simulink model "navion_simulation_Gramajo_yaw_rate_feedback"  (Simulink 8.7)
settings: Solver=ode45  StartTime=0.0  StopTime=20  MaxStep=0.1  RelTol=1e-3
PreLoadFcn:
  | aero1=datcomimport('NavionOut.out');
  | load bank_turn.mat
  | load elevator.mat
  | modify
values from neighbouring files (symbols this model uses):
  aileron = [-45 -40 -35 -30 -25 -20 -15 -10 -5 0 5 10 ... (19 elements, 1x19)]    [bank_turn.mat]    (also in calc_bank_turn.m = -45:5:45)
  delCl = [-0.189280957379 -0.179943445881 -0.170605934382 -0.161268422884 -0.151930911386 -0.142593399888 -0.13325588839 -0.123918376892 -0.114580865393 -0.105243353895 -0.0959058423971 -0.0865683308989 ... (361 elements, 19x19)]    [bank_turn.mat]
  delCn = [0.0592975613365 0.0530143760293 0.0467311907221 0.040448005415 0.0341648201078 0.0278816348006 0.0215984494934 0.0153152641863 0.00903207887907 0.00274889357189 -0.00353429173529 -0.00981747704247 ... (361 elements, 19x19)]    [bank_turn.mat]
  delCy = [-0.123307511653 -0.109606677025 -0.0959058423971 -0.0822050077689 -0.0685041731408 -0.0548033385126 -0.0411025038845 -0.0274016692563 -0.0137008346282 0 0.0137008346282 0.0274016692563 ... (19 elements, 1x19)]    [bank_turn.mat]
  dt = 5    [search_and_coverage.m]    (also in search_and_coverage_multiple_turn_durations.m = Turn_durations(ii); search_and_coverage_time_constraint.m = 13)
  rudder = [-45 -40 -35 -30 -25 -20 -15 -10 -5 0 5 10 ... (19 elements, 1x19)]    [bank_turn.mat]    (also in calc_bank_turn.m = -45:5:45)
  V_mass = 5    [search_and_coverage.m]    (also in search_and_coverage_multiple_turn_durations.m; search_and_coverage_time_constraint.m)
  Velocity = vel    [RHC_opt.m]    (also in RHC_opt_mod_algo.m; search_and_coverage.m = sqrt(2*Weight/(rho*W_area)*(1/CL)); search_and_coverage_multiple_turn_durations.m = sqrt(2*Weight/(rho*W_area)*(1/CL)); search_and_coverage_time_constraint.m = sqrt(2*Weight/(rho*W_area)*(1/CL)))
undefined symbols (not defined in the file or in its folder): alpha_table, delCD, delCL, delCm, delE, desired_omega
libraries: aerolibasang x4, simulink x3, aerolibtransform2 x2, aerolib6dof2 x1, aerolibatmos2 x1, aerolibadyn x1, aerolibutil x1
settings Model: Creator=ggramajo  LastModifiedBy=ggramajo
settings DataIOCC: LimitDataPoints=off  SaveFormat=Structure
settings DebuggingCC: AlgebraicLoopMsg=none  UnderspecifiedInitializationDetection=Simplified  MergeDetectMultiDrivingBlocksExec=error
settings HardwareCC: ProdBitPerPointer=64  ProdLargestAtomicFloat=Float  ProdIntDivRoundTo=Zero  ProdEndianess=LittleEndian  ProdWordSize=64  ProdHWDeviceType=Intel->x86-64 (Windows64)
settings ModelReferenceCC: PropagateSignalLabelsOutOfModel=on
settings ConfigComp: CovModelRefEnable=off

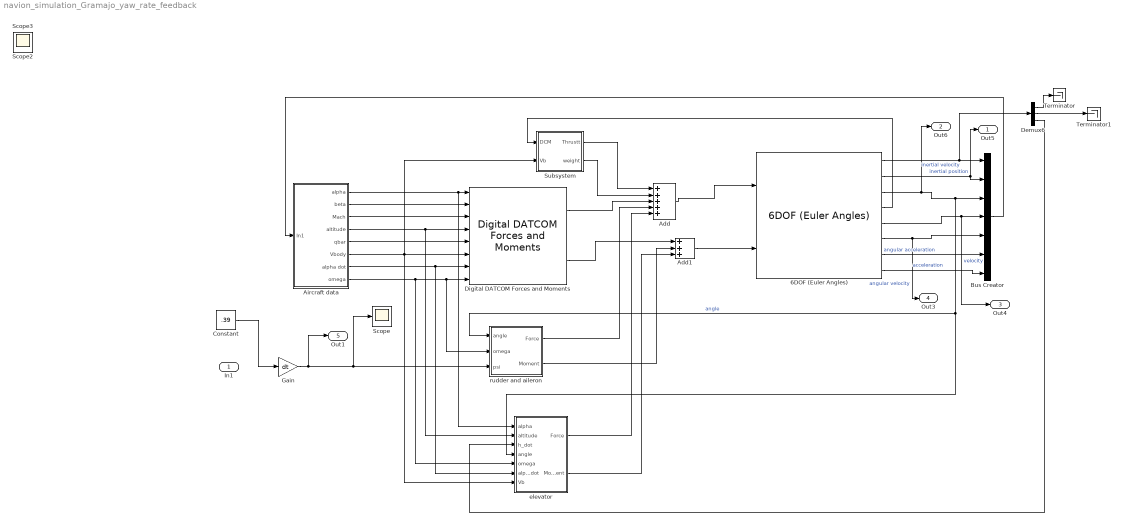
== system navion_simulation_Gramajo_yaw_rate_feedback ==
  In1 : Inport
  6DOF (Euler Angles) : aerolib6dof2/6DOF (Euler Angles)  units=Metric (MKS)  mtype=Fixed  rep=Euler Angles  xme_0=[0 0 -121]  Vm_0=[28 0 0]  eul_0=[0 0 0]  pm_0=[0 0 0]  mass_0=V_mass  mass_e=0.5  mass_f=2.0  inertia=[.057 0 0;0 .163 0;0 0 .192]  inertia_e=eye(3)  inertia_f=2*eye(3)  k_quat=1.0  vre_flag=on
  Add : Sum  Inputs=+++++
  Add1 : Sum  Inputs=+++
  "Aircraft data " : Subsystem
  Bus Creator : BusCreator  Inputs=7
  Constant : Constant  Value=.39
  Demux6 : Demux  Outputs=3
  Digital DATCOM Forces and Moments : aerolibadyn/Digital DATCOM Forces and Moments  units=Metric (MKS)  dcase=aero1{1}  fmode=Body  buildno=0  imethod=Linear  emethod=Linear  rmethod=Linear Extrapolation  action=None
  Gain : Gain  Gain=dt
  Scope : Scope
  Subsystem : Subsystem
  Terminator : Terminator
  Terminator1 : Terminator
  elevator : Subsystem
  rudder and aileron : Subsystem
  Out5 : Outport
  Out6 : Outport  Port=2
  Out4 : Outport  Port=3
  Out3 : Outport  Port=4
  Out1 : Outport  Port=5
  Scope2 : Scope
  Scope3 : Scope
  wires:
  "Aircraft data "/3(Mach) -> Digital DATCOM Forces and Moments/3
  "Aircraft data "/5("qbar ") -> Digital DATCOM Forces and Moments/5
  "Aircraft data "/6(Vbody) -> elevator/7(Vb), Subsystem/2("Vb "), Digital DATCOM Forces and Moments/6
  "Aircraft data "/1(alpha) -> elevator/1(alpha), Digital DATCOM Forces and Moments/1
  Add/1 -> 6DOF (Euler Angles)/1
  Add1/1 -> 6DOF (Euler Angles)/2
  6DOF (Euler Angles)/1 -> Demux6/1, Bus Creator/1  "inertial velocity"
  6DOF (Euler Angles)/2 -> Bus Creator/2, Out5/1  "inertial position"
  6DOF (Euler Angles)/3 -> Out6/1, elevator/4(angle), rudder and aileron/1(angle), Bus Creator/3  "angle"
  6DOF (Euler Angles)/5 -> Out4/1, Bus Creator/4  "velocity"
  6DOF (Euler Angles)/6 -> Out3/1, Bus Creator/5  "angular velocity"
  6DOF (Euler Angles)/7 -> Bus Creator/6  "angular acceleration"
  6DOF (Euler Angles)/8 -> Bus Creator/7  "acceleration"
  Bus Creator/1 -> "Aircraft data "/1(In1)
  "Aircraft data "/2(beta) -> Digital DATCOM Forces and Moments/2
  Digital DATCOM Forces and Moments/1 -> Add/3
  "Aircraft data "/7("alpha dot ") -> elevator/6(alpha_dot), Digital DATCOM Forces and Moments/7
  "Aircraft data "/8(omega) -> elevator/5(omega), rudder and aileron/2(omega), Digital DATCOM Forces and Moments/8
  Digital DATCOM Forces and Moments/2 -> Add1/1
  "Aircraft data "/4(altitude) -> elevator/2(altitude), Digital DATCOM Forces and Moments/4
  6DOF (Euler Angles)/4 -> Subsystem/1(DCM)
  Demux6/3 -> elevator/3(h_dot)
  Subsystem/1("Thrustt ") -> Add/1
  Subsystem/2(weight) -> Add/2
  elevator/1(Force) -> Add/5
  elevator/2(Moment) -> Add1/3
  rudder and aileron/1(Force) -> Add/4
  rudder and aileron/2(Moment) -> Add1/2
  Demux6/1 -> Terminator/1
  Demux6/2 -> Terminator1/1
  Gain/1 -> Scope/1, rudder and aileron/3(psi), Out1/1
  Constant/1 -> Gain/1

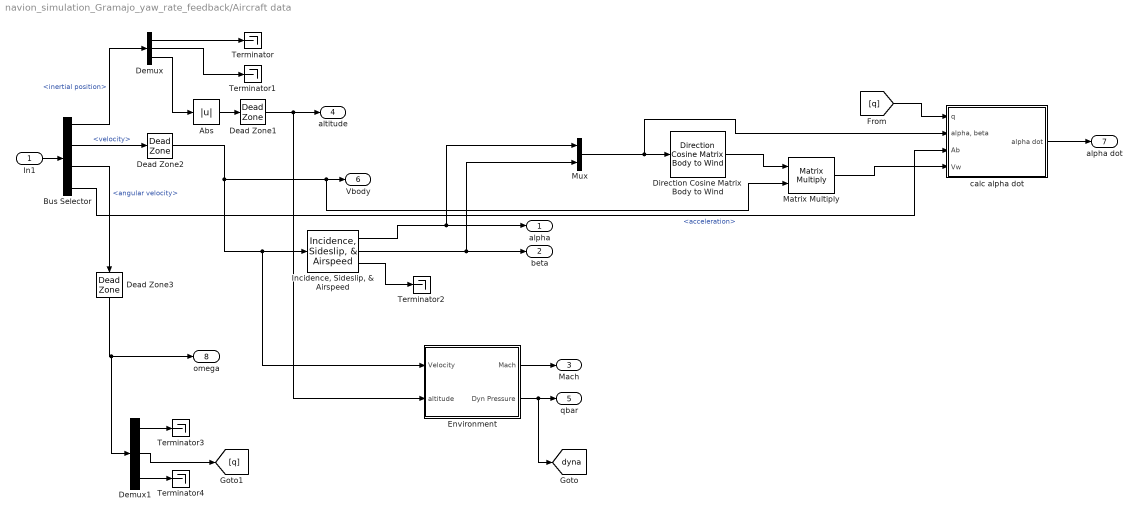
== system navion_simulation_Gramajo_yaw_rate_feedback/Aircraft data  ==
  In1 : Inport
  Abs : Abs
  Bus Selector : BusSelector  OutputSignals=inertial position,velocity,angular velocity,acceleration
  Dead Zone1 : DeadZone  LowerValue=-0.001  UpperValue=0.001  SaturateOnIntegerOverflow=on
  Dead Zone2 : DeadZone  LowerValue=-0.001  UpperValue=0.001  SaturateOnIntegerOverflow=on
  Dead Zone3 : DeadZone  LowerValue=-0.001  UpperValue=0.001  SaturateOnIntegerOverflow=on
  Demux : Demux  Outputs=3
  Demux1 : Demux  Outputs=3
  Direction Cosine Matrix Body to Wind : aerolibtransform2/Direction Cosine Matrix Body to Wind
  Environment : Subsystem
  "Incidence, Sideslip, & Airspeed" : aerolibasang/Incidence, Sideslip, & Airspeed
  Matrix Multiply : Product  Multiplication=Matrix(*)
  Mux : Mux  Inputs=2
  Terminator{,1..4} (5 alike) : Terminator
  calc alpha dot : Subsystem
  alpha : Outport
  beta : Outport  Port=2
  Mach : Outport  Port=3
  altitude : Outport  Port=4
  "qbar " : Outport  Port=5
  Vbody : Outport  Port=6
  "alpha dot " : Outport  Port=7
  omega : Outport  Port=8
  tag scope: dyna=global
  wires:
  In1/1 -> Bus Selector/1
  Bus Selector/1 -> Demux/1  "<inertial position>"
  Demux/1 -> Terminator/1
  Demux/3 -> Abs/1
  Demux/2 -> Terminator1/1
  Bus Selector/2 -> Dead Zone2/1  "<velocity>"
  "Incidence, Sideslip, & Airspeed"/1 -> Mux/1, alpha/1
  "Incidence, Sideslip, & Airspeed"/2 -> Mux/2, beta/1
  "Incidence, Sideslip, & Airspeed"/3 -> Terminator2/1
  Dead Zone1/1 -> Environment/2(altitude), altitude/1
  Abs/1 -> Dead Zone1/1
  Environment/1(Mach) -> Mach/1
  Environment/2(Dyn Pressure) -> [dyna], "qbar "/1
  Mux/1 -> calc alpha dot/2("alpha, beta"), Direction Cosine Matrix Body to Wind/1
  Bus Selector/3 -> Dead Zone3/1  "<angular velocity>"
  Direction Cosine Matrix Body to Wind/1 -> Matrix Multiply/1
  Bus Selector/4 -> calc alpha dot/3("Ab ")  "<acceleration>"
  [q] -> calc alpha dot/1("q ")
  Demux1/1 -> Terminator3/1
  Demux1/2 -> [q]
  calc alpha dot/1("alpha dot ") -> "alpha dot "/1
  Matrix Multiply/1 -> calc alpha dot/4("Vw ")
  Demux1/3 -> Terminator4/1
  Dead Zone2/1 -> Environment/1("Velocity "), "Incidence, Sideslip, & Airspeed"/1, Matrix Multiply/2, Vbody/1
  Dead Zone3/1 -> omega/1, Demux1/1

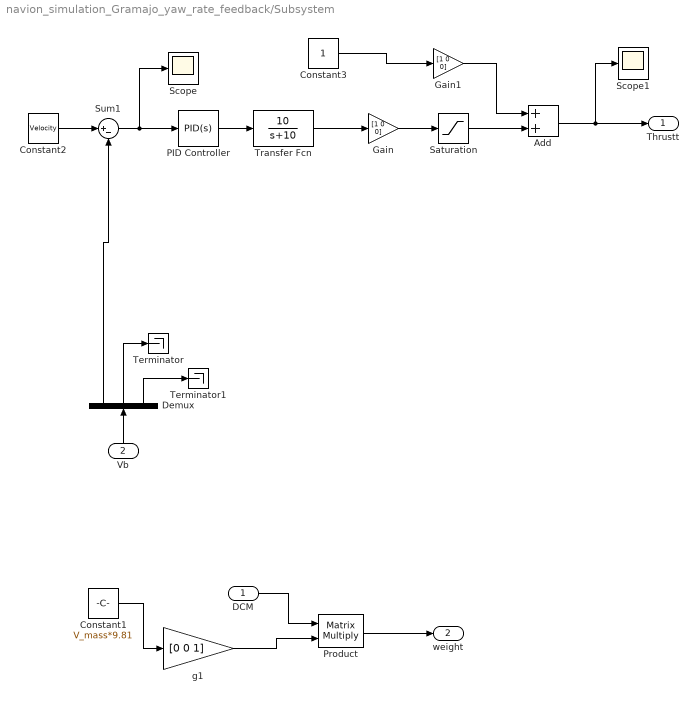
== system navion_simulation_Gramajo_yaw_rate_feedback/Subsystem ==
  DCM : Inport
  "Vb " : Inport  Port=2
  Add : Sum
  Constant1 : Constant  Value=V_mass*9.81
  Constant2 : Constant  Value=Velocity
  Constant3 : Constant
  Demux : Demux  Outputs=3
  Gain : Gain  Gain=[1 0 0]
  Gain1 : Gain  Gain=[1 0 0]
  PID Controller : simulink/Continuous/PID Controller  Controller=PID  TimeDomain=Continuous-time  SampleTime=-1  IntegratorMethod=Forward Euler  FilterMethod=Forward Euler  Form=Parallel  UseFilter=on  ControllerParametersSource=internal  P=1378.85680869118  I=7872.63938553885  D=41.0333927112897  N=486.626215957967  InitialConditionSource=internal  InitialConditionForIntegrator=0  InitialConditionForFilter=0  ExternalReset=none  LimitOutput=off  UpperSaturationLimit=inf  LowerSaturationLimit=-inf  LinearizeAsGain=on  AntiWindupMode=none  Kb=1  TrackingMode=off  Kt=1  PParamMin=[]  PParamMax=[]  IParamMin=[]  IParamMax=[]  DParamMin=[]  DParamMax=[]  NParamMin=[]  NParamMax=[]  KbParamMin=[]  KbParamMax=[]  KtParamMin=[]  KtParamMax=[]  POutMin=[]  POutMax=[]  IOutMin=[]  IOutMax=[]  DOutMin=[]  DOutMax=[]  NOutMin=[]  NOutMax=[]  KbOutMin=[]  KbOutMax=[]  KtOutMin=[]  KtOutMax=[]  IntegratorOutMin=[]  IntegratorOutMax=[]  FilterOutMin=[]  FilterOutMax=[]  SumOutMin=[]  SumOutMax=[]  SumI1OutMin=[]  SumI1OutMax=[]  SumI2OutMin=[]  SumI2OutMax=[]  SumI3OutMin=[]  SumI3OutMax=[]  SumDOutMin=[]  SumDOutMax=[]  SaturationOutMin=[]  SaturationOutMax=[]  IntegratorContinuousStateAttributes=''  IntegratorStateMustResolveToSignalObject=off  IntegratorRTWStateStorageClass=Auto  FilterContinuousStateAttributes=''  FilterStateMustResolveToSignalObject=off  FilterRTWStateStorageClass=Auto  DifferentiatorICPrevScaledInput=0  DifferentiatorOutMin=[]  DifferentiatorOutMax=[]
  Product : Product  Multiplication=Matrix(*)  SaturateOnIntegerOverflow=on  InputSameDT=on  OutDataTypeStr=Inherit: Same as first input
  Saturation : Saturate  UpperLimit=5  LowerLimit=-1
  Scope : Scope
  Scope1 : Scope
  Sum1 : Sum  Inputs=|+-
  Terminator : Terminator
  Terminator1 : Terminator
  Transfer Fcn : TransferFcn  Numerator=[10]  Denominator=[1 10]
  g1 : Gain  Gain=[0 0 1]  SaturateOnIntegerOverflow=on  OutDataTypeStr=Inherit: Same as input  ParamDataTypeStr=Inherit: Same as input
  "Thrustt " : Outport
  weight : Outport  Port=2
  wires:
  Constant2/1 -> Sum1/1
  "Vb "/1 -> Demux/1
  Demux/2 -> Terminator/1
  Demux/3 -> Terminator1/1
  Transfer Fcn/1 -> Gain/1
  Demux/1 -> Sum1/2
  Sum1/1 -> Scope/1, PID Controller/1
  Constant1/1 -> g1/1
  DCM/1 -> Product/1
  g1/1 -> Product/2
  Product/1 -> weight/1
  PID Controller/1 -> Transfer Fcn/1
  Gain/1 -> Saturation/1
  Constant3/1 -> Gain1/1
  Gain1/1 -> Add/1
  Add/1 -> Scope1/1, "Thrustt "/1
  Saturation/1 -> Add/2

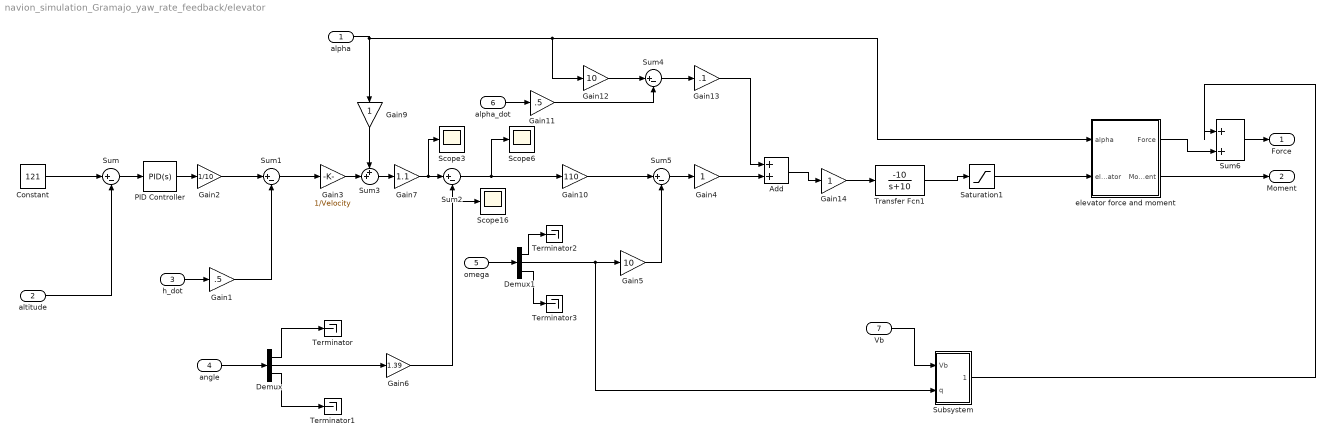
== system navion_simulation_Gramajo_yaw_rate_feedback/elevator ==
  alpha : Inport
  altitude : Inport  Port=2
  h_dot : Inport  Port=3
  angle : Inport  Port=4
  omega : Inport  Port=5
  alpha_dot : Inport  Port=6
  Vb : Inport  Port=7
  Add : Sum
  Constant : Constant  Value=121
  Demux : Demux  Outputs=3
  Demux1 : Demux  Outputs=3
  Gain1 : Gain  Gain=.5
  Gain10 : Gain  Gain=110
  Gain11 : Gain  Gain=.5
  Gain12 : Gain  Gain=10
  Gain13 : Gain  Gain=.1
  Gain14 : Gain
  Gain2 : Gain  Gain=1/10
  Gain3 : Gain  Gain=1/Velocity
  Gain4 : Gain
  Gain5 : Gain  Gain=10
  Gain6 : Gain  Gain=1.39
  Gain7 : Gain  Gain=1.1
  Gain9 : Gain
  PID Controller : simulink/Continuous/PID Controller  Controller=PID  TimeDomain=Continuous-time  SampleTime=-1  IntegratorMethod=Forward Euler  FilterMethod=Forward Euler  Form=Parallel  UseFilter=on  ControllerParametersSource=internal  P=27.8572060055225  I=30.4447135032815  D=6.28354456949659  N=474.535862872723  InitialConditionSource=internal  InitialConditionForIntegrator=0  InitialConditionForFilter=0  ExternalReset=none  LimitOutput=off  UpperSaturationLimit=inf  LowerSaturationLimit=-inf  LinearizeAsGain=on  AntiWindupMode=none  Kb=1  TrackingMode=off  Kt=1  PParamMin=[]  PParamMax=[]  IParamMin=[]  IParamMax=[]  DParamMin=[]  DParamMax=[]  NParamMin=[]  NParamMax=[]  KbParamMin=[]  KbParamMax=[]  KtParamMin=[]  KtParamMax=[]  POutMin=[]  POutMax=[]  IOutMin=[]  IOutMax=[]  DOutMin=[]  DOutMax=[]  NOutMin=[]  NOutMax=[]  KbOutMin=[]  KbOutMax=[]  KtOutMin=[]  KtOutMax=[]  IntegratorOutMin=[]  IntegratorOutMax=[]  FilterOutMin=[]  FilterOutMax=[]  SumOutMin=[]  SumOutMax=[]  SumI1OutMin=[]  SumI1OutMax=[]  SumI2OutMin=[]  SumI2OutMax=[]  SumI3OutMin=[]  SumI3OutMax=[]  SumDOutMin=[]  SumDOutMax=[]  SaturationOutMin=[]  SaturationOutMax=[]  IntegratorContinuousStateAttributes=''  IntegratorStateMustResolveToSignalObject=off  IntegratorRTWStateStorageClass=Auto  FilterContinuousStateAttributes=''  FilterStateMustResolveToSignalObject=off  FilterRTWStateStorageClass=Auto  DifferentiatorICPrevScaledInput=0  DifferentiatorOutMin=[]  DifferentiatorOutMax=[]
  Saturation1 : Saturate  UpperLimit=20  LowerLimit=-30
  Scope16 : Scope
  Scope3 : Scope
  Scope6 : Scope
  Subsystem : Subsystem
  Sum{,1..2,4..5} (5 alike) : Sum  Inputs=|+-
  Sum3 : Sum  Inputs=++|
  Sum6 : Sum  Inputs=|++
  Terminator{,1..3} (4 alike) : Terminator
  Transfer Fcn1 : TransferFcn  Numerator=[-10]  Denominator=[1 10]
  "elevator force and moment " : Subsystem
  Force : Outport
  Moment : Outport  Port=2
  wires:
  "elevator force and moment "/2(Moment) -> Moment/1
  Constant/1 -> Sum/1
  altitude/1 -> Sum/2
  h_dot/1 -> Gain1/1
  Saturation1/1 -> "elevator force and moment "/2(elevator)
  angle/1 -> Demux/1
  Demux/1 -> Terminator/1
  Demux/3 -> Terminator1/1
  omega/1 -> Demux1/1
  Sum5/1 -> Gain4/1
  Gain5/1 -> Sum5/2
  Sum2/1 -> Scope6/1, Gain10/1
  Gain1/1 -> Sum1/2
  Demux/2 -> Gain6/1
  Demux1/1 -> Terminator2/1
  Demux1/3 -> Terminator3/1
  Demux1/2 -> Gain5/1, Subsystem/2(q)
  Gain6/1 -> Scope16/1, Sum2/2
  Gain3/1 -> Sum3/2
  alpha/1 -> Gain12/1, "elevator force and moment "/1(alpha), Gain9/1
  Gain9/1 -> Sum3/1
  Sum1/1 -> Gain3/1
  Transfer Fcn1/1 -> Saturation1/1
  Sum/1 -> PID Controller/1
  Gain2/1 -> Sum1/1
  Gain10/1 -> Sum5/1
  Add/1 -> Gain14/1
  Gain4/1 -> Add/2
  Sum4/1 -> Gain13/1
  alpha_dot/1 -> Gain11/1
  Gain11/1 -> Sum4/2
  Gain12/1 -> Sum4/1
  Gain13/1 -> Add/1
  Gain14/1 -> Transfer Fcn1/1
  Sum3/1 -> Gain7/1
  Gain7/1 -> Scope3/1, Sum2/1
  PID Controller/1 -> Gain2/1
  Vb/1 -> Subsystem/1(Vb)
  Sum6/1 -> Force/1
  "elevator force and moment "/1(Force) -> Sum6/2
  Subsystem/1(CLq) -> Sum6/1

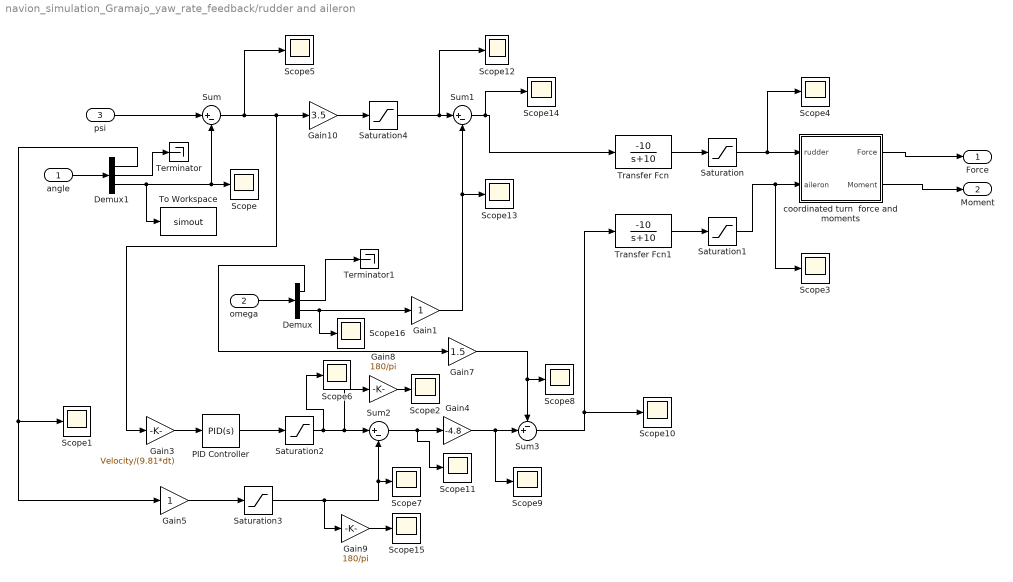
== system navion_simulation_Gramajo_yaw_rate_feedback/rudder and aileron ==
  angle : Inport
  omega : Inport  Port=2
  psi : Inport  Port=3
  Demux : Demux  Outputs=3
  Demux1 : Demux  Outputs=3
  Gain1 : Gain
  Gain10 : Gain  Gain=3.5
  Gain3 : Gain  Gain=Velocity/(9.81*dt)
  Gain4 : Gain  Gain=-4.8
  Gain5 : Gain
  Gain7 : Gain  Gain=1.5
  Gain8 : Gain  Gain=180/pi
  Gain9 : Gain  Gain=180/pi
  PID Controller : simulink/Continuous/PID Controller  Controller=PID  TimeDomain=Continuous-time  SampleTime=-1  IntegratorMethod=Forward Euler  FilterMethod=Forward Euler  Form=Parallel  UseFilter=on  ControllerParametersSource=internal  P=15.0986911644413  I=0.176703988972368  D=3.35005448489008  N=153.250185887762  InitialConditionSource=internal  InitialConditionForIntegrator=0  InitialConditionForFilter=0  ExternalReset=none  LimitOutput=off  UpperSaturationLimit=inf  LowerSaturationLimit=-inf  LinearizeAsGain=on  AntiWindupMode=none  Kb=1  TrackingMode=off  Kt=1  PParamMin=[]  PParamMax=[]  IParamMin=[]  IParamMax=[]  DParamMin=[]  DParamMax=[]  NParamMin=[]  NParamMax=[]  KbParamMin=[]  KbParamMax=[]  KtParamMin=[]  KtParamMax=[]  POutMin=[]  POutMax=[]  IOutMin=[]  IOutMax=[]  DOutMin=[]  DOutMax=[]  NOutMin=[]  NOutMax=[]  KbOutMin=[]  KbOutMax=[]  KtOutMin=[]  KtOutMax=[]  IntegratorOutMin=[]  IntegratorOutMax=[]  FilterOutMin=[]  FilterOutMax=[]  SumOutMin=[]  SumOutMax=[]  SumI1OutMin=[]  SumI1OutMax=[]  SumI2OutMin=[]  SumI2OutMax=[]  SumI3OutMin=[]  SumI3OutMax=[]  SumDOutMin=[]  SumDOutMax=[]  SaturationOutMin=[]  SaturationOutMax=[]  IntegratorContinuousStateAttributes=''  IntegratorStateMustResolveToSignalObject=off  IntegratorRTWStateStorageClass=Auto  FilterContinuousStateAttributes=''  FilterStateMustResolveToSignalObject=off  FilterRTWStateStorageClass=Auto  DifferentiatorICPrevScaledInput=0  DifferentiatorOutMin=[]  DifferentiatorOutMax=[]
  Saturation : Saturate  UpperLimit=15  LowerLimit=-15
  Saturation1 : Saturate  UpperLimit=20  LowerLimit=-20
  Saturation2 : Saturate  UpperLimit=.8411  LowerLimit=-.8411
  Saturation3 : Saturate  UpperLimit=.8411  LowerLimit=-.8411
  Saturation4 : Saturate  UpperLimit=1.5*desired_omega  LowerLimit=-1.5*abs(desired_omega)
  Scope{,1..16} (17 alike) : Scope
  Sum : Sum  Inputs=|+-
  Sum1 : Sum  Inputs=|+-
  Sum2 : Sum  Inputs=|+-
  Sum3 : Sum  Inputs=-+|
  Terminator : Terminator
  Terminator1 : Terminator
  To Workspace : ToWorkspace  VariableName=simout  SaveFormat=Structure With Time  SampleTime=-1
  Transfer Fcn : TransferFcn  Numerator=[-10]  Denominator=[1 10]
  Transfer Fcn1 : TransferFcn  Numerator=[-10]  Denominator=[1 10]
  "coordinated turn  force and moments  " : Subsystem
  Force : Outport
  Moment : Outport  Port=2
  wires:
  "coordinated turn  force and moments  "/1(Force) -> Force/1
  "coordinated turn  force and moments  "/2(Moment) -> Moment/1
  Transfer Fcn/1 -> Saturation/1
  Saturation/1 -> Scope4/1, "coordinated turn  force and moments  "/1(rudder)
  omega/1 -> Demux/1
  angle/1 -> Demux1/1
  Demux1/3 -> To Workspace/1, Scope/1, Sum/2
  Saturation1/1 -> Scope3/1, "coordinated turn  force and moments  "/2(aileron)
  Sum3/1 -> Scope10/1, Transfer Fcn1/1
  Sum1/1 -> Scope14/1, Transfer Fcn/1
  Demux1/1 -> Scope1/1, Gain5/1
  Demux1/2 -> Terminator/1
  Sum2/1 -> Scope11/1, Gain4/1
  Gain5/1 -> Saturation3/1
  PID Controller/1 -> Saturation2/1
  Demux/1 -> Gain7/1
  Gain4/1 -> Scope9/1, Sum3/2
  Gain7/1 -> Scope8/1, Sum3/1
  Transfer Fcn1/1 -> Saturation1/1
  Demux/2 -> Terminator1/1
  Gain3/1 -> PID Controller/1
  Sum/1 -> Gain3/1, Gain10/1, Scope5/1
  psi/1 -> Sum/1
  Gain1/1 -> Scope13/1, Sum1/2
  Gain8/1 -> Scope2/1
  Saturation2/1 -> Scope6/1, Gain8/1, Sum2/1
  Gain9/1 -> Scope15/1
  Saturation3/1 -> Gain9/1, Scope7/1, Sum2/2
  Demux/3 -> Gain1/1, Scope16/1
  Gain10/1 -> Saturation4/1
  Saturation4/1 -> Scope12/1, Sum1/1

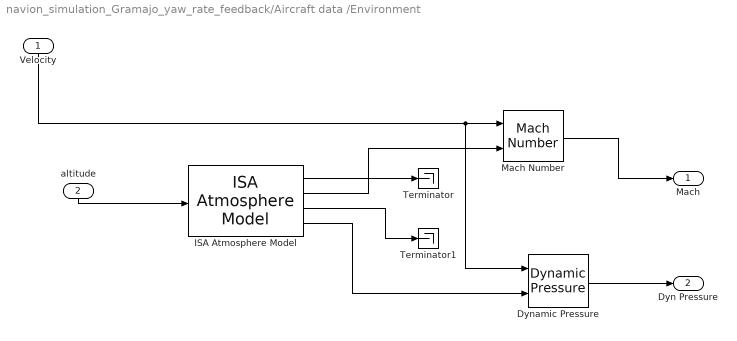
== system navion_simulation_Gramajo_yaw_rate_feedback/Aircraft data /Environment ==
  "Velocity " : Inport
  altitude : Inport  Port=2
  Dynamic Pressure : aerolibasang/Dynamic Pressure
  ISA Atmosphere Model : aerolibatmos2/ISA Atmosphere Model  custom=off  g=9.80665  gamma=1.4  R=287.0531  L=0.0065  h_trop=11000  h_strat=20000  rho0=1.225  P0=101325  T0=288.15  h0=0
  Mach Number : aerolibasang/Mach Number
  Terminator : Terminator
  Terminator1 : Terminator
  Mach : Outport
  Dyn Pressure : Outport  Port=2
  wires:
  Mach Number/1 -> Mach/1
  altitude/1 -> ISA Atmosphere Model/1
  ISA Atmosphere Model/2 -> Mach Number/2
  ISA Atmosphere Model/4 -> Dynamic Pressure/2
  ISA Atmosphere Model/1 -> Terminator/1
  ISA Atmosphere Model/3 -> Terminator1/1
  "Velocity "/1 -> Dynamic Pressure/1, Mach Number/1
  Dynamic Pressure/1 -> Dyn Pressure/1

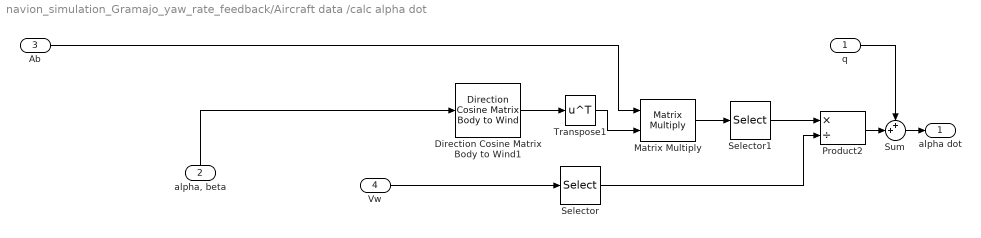
== system navion_simulation_Gramajo_yaw_rate_feedback/Aircraft data /calc alpha dot ==
  "q " : Inport
  "alpha, beta" : Inport  Port=2
  "Ab " : Inport  Port=3
  "Vw " : Inport  Port=4
  Direction Cosine Matrix Body to Wind1 : aerolibtransform2/Direction Cosine Matrix Body to Wind
  Matrix Multiply : Product  Multiplication=Matrix(*)
  Product2 : Product  Inputs=*/  SaturateOnIntegerOverflow=on  InputSameDT=on  OutDataTypeStr=Inherit: Same as first input
  Selector : Selector  InputPortWidth=3  IndexOptions=Index vector (dialog)  Indices=[1]  OutputSizes=1
  Selector1 : Selector  InputPortWidth=3  IndexOptions=Index vector (dialog)  Indices=[3]  OutputSizes=1
  Sum : Sum  Inputs=++|
  Transpose1 : Math  Operator=transpose  SaturateOnIntegerOverflow=on
  "alpha dot " : Outport
  wires:
  "Vw "/1 -> Selector/1
  Direction Cosine Matrix Body to Wind1/1 -> Transpose1/1
  Selector/1 -> Product2/2
  "alpha, beta"/1 -> Direction Cosine Matrix Body to Wind1/1
  Matrix Multiply/1 -> Selector1/1
  Selector1/1 -> Product2/1
  Sum/1 -> "alpha dot "/1
  Product2/1 -> Sum/2
  "q "/1 -> Sum/1
  "Ab "/1 -> Matrix Multiply/1
  Transpose1/1 -> Matrix Multiply/2

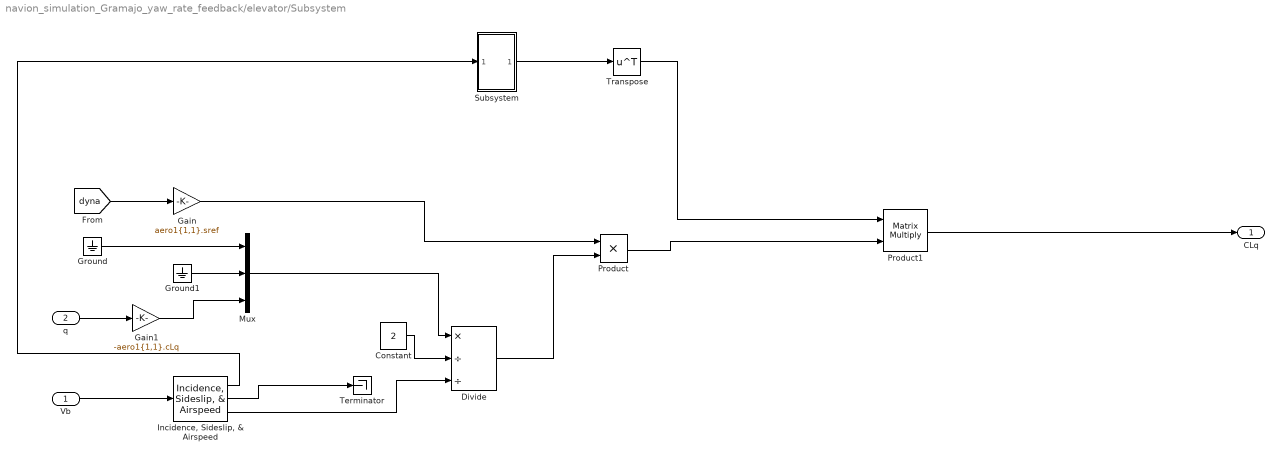
== system navion_simulation_Gramajo_yaw_rate_feedback/elevator/Subsystem ==
  Vb : Inport
  q : Inport  Port=2
  Constant : Constant  Value=2
  Divide : Product  Inputs=*//
  Gain : Gain  Gain=aero1{1,1}.sref
  Gain1 : Gain  Gain=-aero1{1,1}.cLq
  Ground : Ground
  Ground1 : Ground
  "Incidence, Sideslip, & Airspeed" : aerolibasang/Incidence, Sideslip, & Airspeed
  Mux : Mux  Inputs=3
  Product : Product
  Product1 : Product  Multiplication=Matrix(*)
  Subsystem : Subsystem
  Terminator : Terminator
  Transpose : Math  Operator=transpose  SaturateOnIntegerOverflow=on
  CLq : Outport
  wires:
  [dyna] -> Gain/1
  q/1 -> Gain1/1
  Vb/1 -> "Incidence, Sideslip, & Airspeed"/1
  "Incidence, Sideslip, & Airspeed"/2 -> Terminator/1
  "Incidence, Sideslip, & Airspeed"/1 -> Subsystem/1(alph)
  "Incidence, Sideslip, & Airspeed"/3 -> Divide/3
  Constant/1 -> Divide/2
  Gain/1 -> Product/1
  Divide/1 -> Product/2
  Gain1/1 -> Mux/3
  Mux/1 -> Divide/1
  Ground/1 -> Mux/1
  Ground1/1 -> Mux/2
  Product/1 -> Product1/2
  Subsystem/1(Out1) -> Transpose/1
  Transpose/1 -> Product1/1
  Product1/1 -> CLq/1

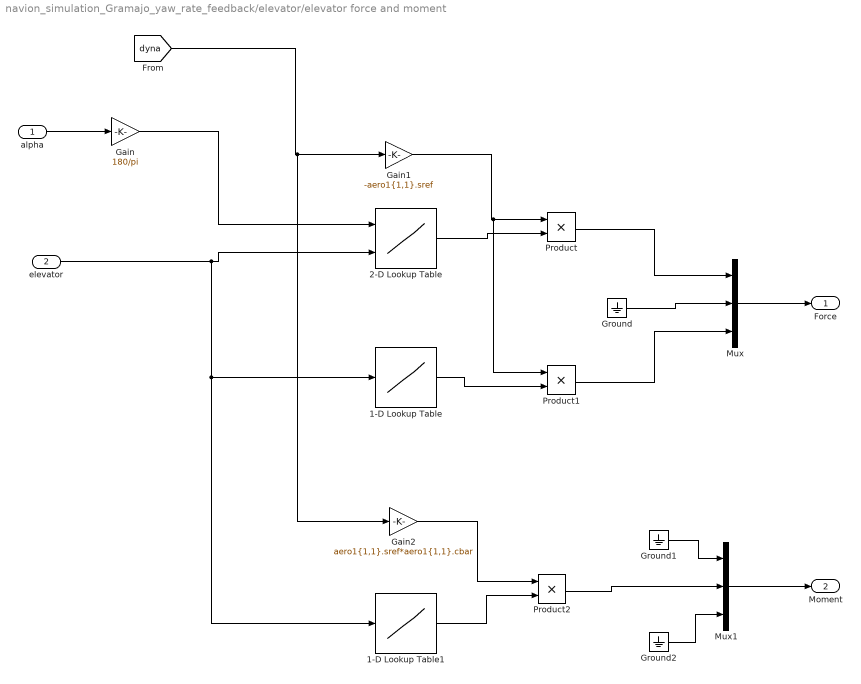
== system navion_simulation_Gramajo_yaw_rate_feedback/elevator/elevator force and moment  ==
  alpha : Inport
  elevator : Inport  Port=2
  1-D Lookup Table : Lookup_n-D  NumberOfTableDimensions=1  BreakpointsForDimension1=delE  Table=delCL  InternalRulePriority=Speed  RndMeth=Simplest  InputSameDT=on
  1-D Lookup Table1 : Lookup_n-D  NumberOfTableDimensions=1  BreakpointsForDimension1=delE  Table=delCm  InternalRulePriority=Speed  RndMeth=Simplest  InputSameDT=on
  2-D Lookup Table : Lookup_n-D  BreakpointsForDimension1=alpha_table  BreakpointsForDimension2=delE  Table=delCD  InternalRulePriority=Speed  RndMeth=Simplest  InputSameDT=on
  Gain : Gain  Gain=180/pi
  Gain1 : Gain  Gain=-aero1{1,1}.sref
  Gain2 : Gain  Gain=aero1{1,1}.sref*aero1{1,1}.cbar
  Ground : Ground
  Ground1 : Ground
  Ground2 : Ground
  Mux : Mux  Inputs=3
  Mux1 : Mux  Inputs=3
  Product : Product
  Product1 : Product
  Product2 : Product
  Force : Outport
  Moment : Outport  Port=2
  wires:
  Gain/1 -> 2-D Lookup Table/1
  alpha/1 -> Gain/1
  2-D Lookup Table/1 -> Product/2
  Gain1/1 -> Product1/1, Product/1
  elevator/1 -> 1-D Lookup Table1/1, 1-D Lookup Table/1, 2-D Lookup Table/2
  [dyna] -> Gain2/1, Gain1/1
  1-D Lookup Table/1 -> Product1/2
  Product/1 -> Mux/1
  Product1/1 -> Mux/3
  Ground/1 -> Mux/2
  Mux/1 -> Force/1
  1-D Lookup Table1/1 -> Product2/2
  Gain2/1 -> Product2/1
  Product2/1 -> Mux1/2
  Ground1/1 -> Mux1/1
  Ground2/1 -> Mux1/3
  Mux1/1 -> Moment/1

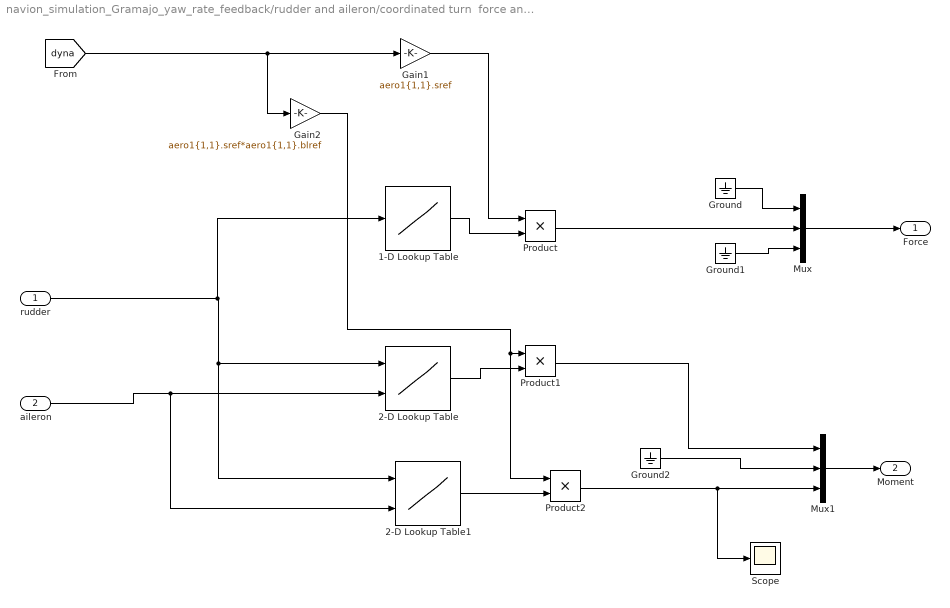
== system navion_simulation_Gramajo_yaw_rate_feedback/rudder and aileron/coordinated turn  force and moments   ==
  rudder : Inport
  aileron : Inport  Port=2
  1-D Lookup Table : Lookup_n-D  NumberOfTableDimensions=1  BreakpointsForDimension1=rudder  Table=delCy  InternalRulePriority=Speed  RndMeth=Simplest  InputSameDT=on
  2-D Lookup Table : Lookup_n-D  BreakpointsForDimension1=rudder  BreakpointsForDimension2=aileron  Table=delCl  InternalRulePriority=Speed  RndMeth=Simplest  InputSameDT=on
  2-D Lookup Table1 : Lookup_n-D  BreakpointsForDimension1=rudder  BreakpointsForDimension2=aileron  Table=delCn  InternalRulePriority=Speed  RndMeth=Simplest  InputSameDT=on
  Gain1 : Gain  Gain=aero1{1,1}.sref
  Gain2 : Gain  Gain=aero1{1,1}.sref*aero1{1,1}.blref
  Ground : Ground
  Ground1 : Ground
  Ground2 : Ground
  Mux : Mux  Inputs=3
  Mux1 : Mux  Inputs=3
  Product : Product
  Product1 : Product
  Product2 : Product
  Scope : Scope
  Force : Outport
  Moment : Outport  Port=2
  wires:
  [dyna] -> Gain2/1, Gain1/1
  Gain1/1 -> Product/1
  1-D Lookup Table/1 -> Product/2
  Product/1 -> Mux/2
  Ground/1 -> Mux/1
  Ground1/1 -> Mux/3
  Mux/1 -> Force/1
  rudder/1 -> 1-D Lookup Table/1, 2-D Lookup Table1/1, 2-D Lookup Table/1
  Gain2/1 -> Product2/1, Product1/1
  aileron/1 -> 2-D Lookup Table1/2, 2-D Lookup Table/2
  2-D Lookup Table1/1 -> Product2/2
  Product1/1 -> Mux1/1
  Product2/1 -> Scope/1, Mux1/3
  Ground2/1 -> Mux1/2
  Mux1/1 -> Moment/1
  2-D Lookup Table/1 -> Product1/2

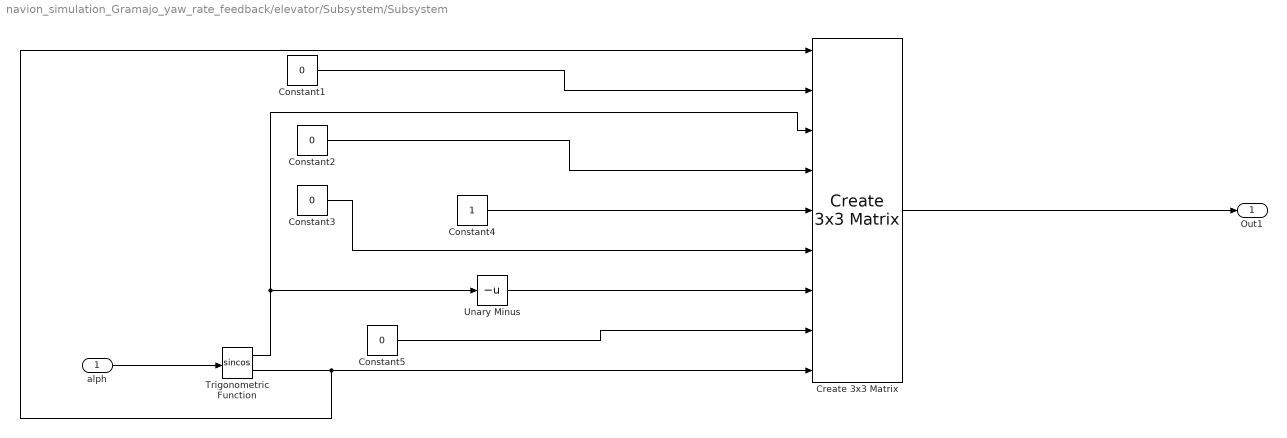
== system navion_simulation_Gramajo_yaw_rate_feedback/elevator/Subsystem/Subsystem ==
  alph : Inport
  Constant{1..3,5} (4 alike) : Constant  Value=0
  Constant4 : Constant
  Create 3x3 Matrix : aerolibutil/Create 3x3 Matrix
  Trigonometric Function : Trigonometry  Operator=sincos
  Unary Minus : UnaryMinus
  Out1 : Outport
  wires:
  Constant1/1 -> Create 3x3 Matrix/2
  Constant2/1 -> Create 3x3 Matrix/4
  Trigonometric Function/1 -> Unary Minus/1, Create 3x3 Matrix/3
  Create 3x3 Matrix/1 -> Out1/1
  alph/1 -> Trigonometric Function/1
  Constant3/1 -> Create 3x3 Matrix/6
  Trigonometric Function/2 -> Create 3x3 Matrix/1, Create 3x3 Matrix/9
  Constant4/1 -> Create 3x3 Matrix/5
  Constant5/1 -> Create 3x3 Matrix/8
  Unary Minus/1 -> Create 3x3 Matrix/7
